simulink model "w1q4"  (R2019b)
settings: Solver=VariableStepAuto  StartTime=0.0  StopTime=10.0  RelTol=1e-3
settings Model: Creator=Vinayak  LastModifiedBy=Vinayak

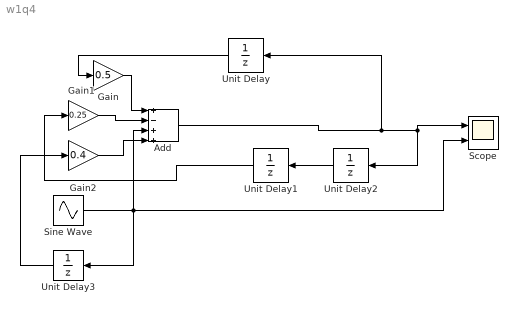
== system w1q4 ==
  Add : Sum  Inputs=+-++
  Gain : Gain  Gain=0.5
  Gain1 : Gain  Gain=0.25
  Gain2 : Gain  Gain=0.4
  Scope : Scope  NumInputPorts=2
  Sine Wave : Sin  SampleTime=0
  Unit Delay{,1..3} (4 alike) : UnitDelay  SampleTime=-1  HasFrameUpgradeWarning=on
  wires:
  Gain/1 -> Add/1
  Gain1/1 -> Add/2
  Gain2/1 -> Add/4
  Add/1 -> Unit Delay/1, Unit Delay2/1, Scope/1
  Unit Delay/1 -> Gain/1
  Unit Delay2/1 -> Unit Delay1/1
  Unit Delay1/1 -> Gain1/1
  Unit Delay3/1 -> Gain2/1
  Sine Wave/1 -> Scope/2, Add/3, Unit Delay3/1
